simulink library "Friction_Compensator_Lib"  (R2014b)
settings: Solver=ode45  StartTime=0.0  StopTime=10.0  RelTol=1e-3
undefined symbols (not defined in the file or in its folder): Ts
settings Model: Creator=xingye  LastModifiedBy=xingye

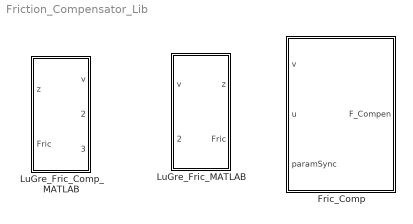
== system Friction_Compensator_Lib ==
  Fric_Comp : Subsystem
  LuGre_Fric_Comp_MATLAB : Subsystem
  LuGre_Fric_MATLAB : Subsystem

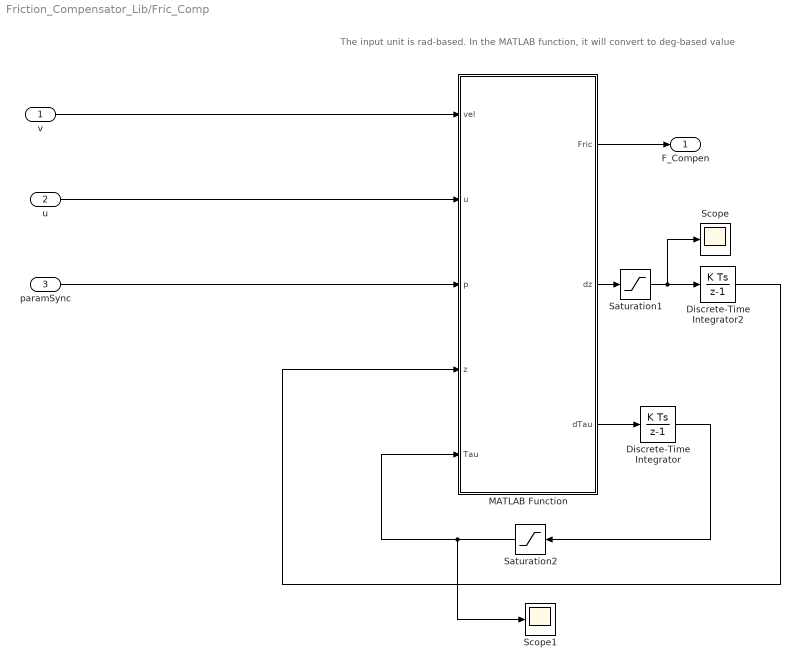
== system Friction_Compensator_Lib/Fric_Comp ==
  note: The input unit is rad-based. In the MATLAB function, it will convert to deg-based value
  v : Inport
  u : Inport  Port=2
  paramSync : Inport  Port=3
  Discrete-Time Integrator : DiscreteIntegrator  SampleTime=Ts
  Discrete-Time Integrator2 : DiscreteIntegrator  InitialConditionSetting=State (most efficient)  SampleTime=Ts
  MATLAB Function : MATLAB Function  TreatAsAtomicUnit=on
  Saturation1 : Saturate  UpperLimit=100  LowerLimit=-100
  Saturation2 : Saturate  UpperLimit=10  LowerLimit=-10
  Scope : Scope
      settings: YMin=-6  YMax=6  SaveName=ScopeData23
  Scope1 : Scope
      settings: SaveName=ScopeData24
  F_Compen : Outport
  wires:
  Saturation2/1 -> MATLAB Function/5(Tau), Scope1/1
  Saturation1/1 -> Discrete-Time Integrator2/1, Scope/1
  Discrete-Time Integrator/1 -> Saturation2/1
  Discrete-Time Integrator2/1 -> MATLAB Function/4(z)
  MATLAB Function/3(dTau) -> Discrete-Time Integrator/1
  MATLAB Function/1(Fric) -> F_Compen/1
  u/1 -> MATLAB Function/2(u)
  MATLAB Function/2(dz) -> Saturation1/1
  v/1 -> MATLAB Function/1(vel)
  paramSync/1 -> MATLAB Function/3(p)

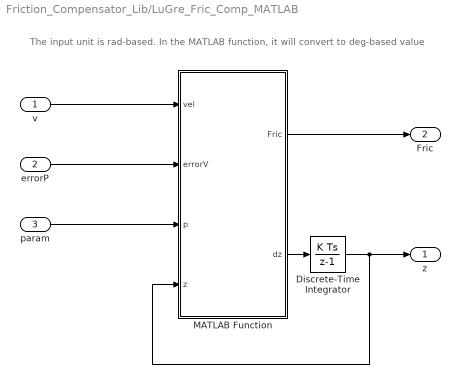
== system Friction_Compensator_Lib/LuGre_Fric_Comp_MATLAB ==
  note: The input unit is rad-based. In the MATLAB function, it will convert to deg-based value
  v : Inport
  errorP : Inport  Port=2
  param : Inport  Port=3
  Discrete-Time Integrator : DiscreteIntegrator  InitialConditionSetting=State (most efficient)  SampleTime=Ts
  MATLAB Function : MATLAB Function  TreatAsAtomicUnit=on
  z : Outport
  Fric : Outport  Port=2
  wires:
  MATLAB Function/2(dz) -> Discrete-Time Integrator/1
  Discrete-Time Integrator/1 -> MATLAB Function/4(z), z/1
  MATLAB Function/1(Fric) -> Fric/1
  v/1 -> MATLAB Function/1(vel)
  param/1 -> MATLAB Function/3(p)
  errorP/1 -> MATLAB Function/2(errorV)

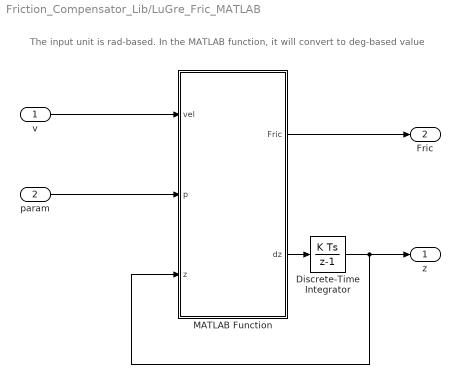
== system Friction_Compensator_Lib/LuGre_Fric_MATLAB ==
  note: The input unit is rad-based. In the MATLAB function, it will convert to deg-based value
  v : Inport
  param : Inport  Port=2
  Discrete-Time Integrator : DiscreteIntegrator  InitialConditionSetting=State (most efficient)  SampleTime=Ts
  MATLAB Function : MATLAB Function  TreatAsAtomicUnit=on
  z : Outport
  Fric : Outport  Port=2
  wires:
  param/1 -> MATLAB Function/2(p)
  v/1 -> MATLAB Function/1(vel)
  MATLAB Function/1(Fric) -> Fric/1
  Discrete-Time Integrator/1 -> z/1, MATLAB Function/3(z)
  MATLAB Function/2(dz) -> Discrete-Time Integrator/1

== matlab function Friction_Compensator_Lib/LuGre_Fric_MATLAB/MATLAB Function ==
  data: vel input; p input; Fric output; z input; dz output
function [Fric,dz] = LuGre_Fric_MATLAB(vel,p,z)
%#codegen

% J = p(1);
alpha0 = p(2);
alpha0v2 = p(3);
alpha1 = p(4);
alpha1v2 = p(5);
alpha2 = p(6);
alpha2v2 = p(7);
alpha3 = p(8); 
alpha3v2 = p(9);
v0 = p(10);
v0v2 = p(11);
sigma0 = p(12);
sigma1 = p(13);
fConst = p(14);

x2 = vel*180/pi;
g = (alpha0+alpha1*exp(-(x2/v0).^2))*(x2>=0)+(alpha0v2+alpha1v2*exp(-(x2/v0v2).^2))*(x2<0);
dz = x2-sigma0/g*abs(x2)*z;

Fric = sigma0*z+sigma1*dz+(alpha2*x2)*(x2>=0)+(abs(alpha2v2)*x2)*(x2<0)+(alpha3*x2^2)*(x2>=0)+(-abs(alpha3v2)*x2^2)*(x2<0)+fConst;

== matlab function Friction_Compensator_Lib/Fric_Comp/MATLAB Function ==
  data: vel input; u input; p input; Fric output; z input; dz output; Tau input; dTau output
function [Fric,dz,dTau] = LuGre_Fric_MATLAB(vel,u,p,z,Tau)
%#codegen

J = p(1);
alpha0 = p(2);
alpha0v2 = p(3);
alpha1 = p(4);
alpha1v2 = p(5);
alpha2 = p(6);
alpha2v2 = p(7);
alpha3 = p(8); 
alpha3v2 = p(9);
v0 = p(10);
v0v2 = p(11);
sigma0 = p(12);
sigma1 = p(13);
fConst = p(14);

L = 4;
u_J = u/(J*180/pi);
dTau = u_J + L*(vel-Tau);
% dTau = u_J;

x2 = Tau*180/pi;
% x2 = vel*180/pi;
g = (alpha0+alpha1*exp(-(x2/v0).^2))*(x2>=0)+(alpha0v2+alpha1v2*exp(-(x2/v0v2).^2))*(x2<0);
dz = -sigma0/g*abs(x2)*z+x2;

Fric = sigma0*z+sigma1*dz+(alpha2*x2)*(x2>=0)+(abs(alpha2v2)*x2)*(x2<0)+(alpha3*x2^2)*(x2>=0)+(-abs(alpha3v2)*x2^2)*(x2<0)+fConst;

== matlab function Friction_Compensator_Lib/LuGre_Fric_Comp_MATLAB/MATLAB Function ==
  data: vel input; errorV input; p input; Fric output; z input; dz output
function [Fric,dz] = LuGre_Fric_MATLAB(vel,errorV,p,z)
%#codegen

% J = p(1);
alpha0 = p(2);
alpha0v2 = p(3);
alpha1 = p(4);
alpha1v2 = p(5);
alpha2 = p(6);
alpha2v2 = p(7);
alpha3 = p(8); 
alpha3v2 = p(9);
v0 = p(10);
v0v2 = p(11);
sigma0 = p(12);
sigma1 = p(13);
fConst = p(14);

% x2 = vel*180/pi;
x2 = (vel+errorV)*180/pi;
g = (alpha0+alpha1*exp(-(x2/v0).^2))*(x2>=0)+(alpha0v2+alpha1v2*exp(-(x2/v0v2).^2))*(x2<0);
dz = -sigma0/g*abs(x2)*z+x2;


Fric = sigma0*z+sigma1*dz+(alpha2*x2)*(x2>=0)+(abs(alpha2v2)*x2)*(x2<0)+(alpha3*x2^2)*(x2>=0)+(-abs(alpha3v2)*x2^2)*(x2<0)+fConst;
